simulink model "Bicycle_model"  (R2024b)
settings: Solver=VariableStepAuto  StartTime=0.0  StopTime=10  RelTol=1e-3
undefined symbols (not defined in the file): Af, Cd, Cl, Cr, g, GR, h_cg, Jf, Jr, M_sprung, Mv, r, rho, wb
libraries: simulink x1
settings Model: Creator=kanishka  LastModifiedBy=kanishka
settings DebuggingCC: AlgebraicLoopMsg=none

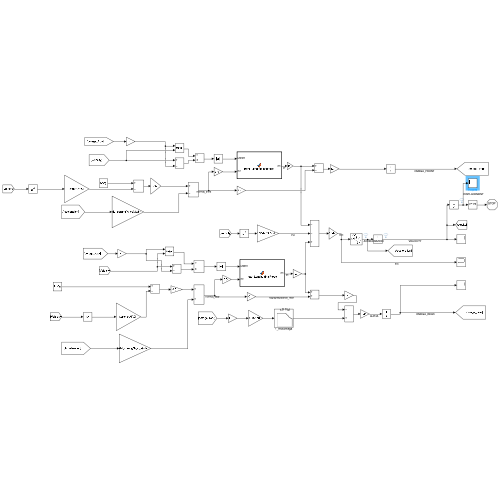
[thumbnail: Simulink's stored preview of the top-level diagram]
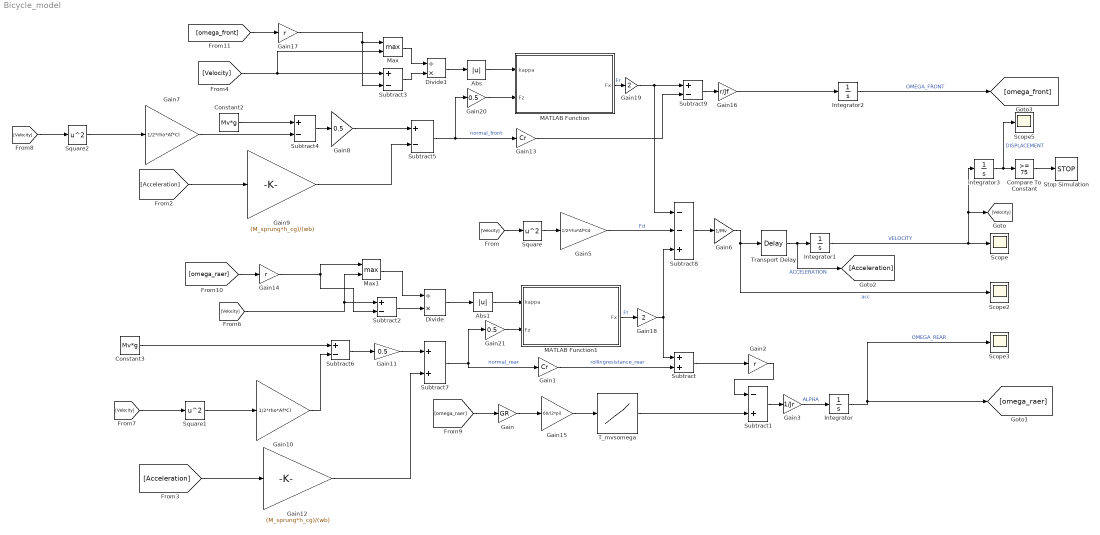
== system Bicycle_model ==
  Abs : Abs  SaturateOnIntegerOverflow=off
  Abs1 : Abs  SaturateOnIntegerOverflow=off
  Compare To Constant : simulink/Logic and Bit Operations/Compare To Constant  relop=>=  const=75  OutDataTypeStr=boolean
  Constant2 : Constant  Value=Mv*g
  Constant3 : Constant  Value=Mv*g
  Divide : Product  Inputs=/*
  Divide1 : Product  Inputs=/*
  Gain : Gain  Gain=GR
  Gain1 : Gain  Gain=Cr
  Gain10 : Gain  Gain=1/2*rho*Af*Cl
  Gain{8,11,20..21} (4 alike) : Gain  Gain=0.5
  Gain12 : Gain  Gain=(M_sprung*h_cg)/(wb)
  Gain13 : Gain  Gain=Cr
  Gain14 : Gain  Gain=r
  Gain15 : Gain  Gain=60/(2*pi)
  Gain16 : Gain  Gain=r/Jf
  Gain17 : Gain  Gain=r
  Gain18 : Gain  Gain=2
  Gain19 : Gain  Gain=2
  Gain2 : Gain  Gain=r
  Gain3 : Gain  Gain=1/Jr
  Gain5 : Gain  Gain=1/2*rho*Af*Cd
  Gain6 : Gain  Gain=1/Mv
  Gain7 : Gain  Gain=1/2*rho*Af*Cl
  Gain9 : Gain  Gain=(M_sprung*h_cg)/(wb)
  Integrator : Integrator  InitialCondition=0.0038455666
  Integrator1 : Integrator  InitialCondition=0.001
  Integrator2 : Integrator  InitialCondition=0.003457549
  Integrator3 : Integrator
  MATLAB Function : MATLAB Function  TreatAsAtomicUnit=on
  MATLAB Function1 : MATLAB Function  TreatAsAtomicUnit=on
  Max : MinMax  Function=max  Inputs=2
  Max1 : MinMax  Function=max  Inputs=2
  Scope{,2..3,5} (4 alike) : Scope
  Square : Math  Operator=square
  Square1 : Math  Operator=square
  Square2 : Math  Operator=square
  Stop Simulation : Stop
  Subtract : Sum
  Subtract1 : Sum  Inputs=-+
  Subtract{2..6,9} (6 alike) : Sum  Inputs=+-
  Subtract7 : Sum
  Subtract8 : Sum  Inputs=--+
  T_mvsomega : Lookup_n-D  NumberOfTableDimensions=1  BreakpointsForDimension1=[1, 3183, 3400, 3600, 3800, 4000, 4200, 4400, 4600, 4800, 5000, 5200, 5400, 5500, 5500.01] ;  Table=[240, 240, 224.653, 212.160, 200.988, 190.985, 181.818, 173.376, 165.571 ,158.408 ,152.788 ,147.016 ,141.381 ,138.991, 0]  InternalRulePriority=Speed  RndMeth=Simplest
  Transport Delay : TransportDelay  DelayTime=0.001  InitialOutput=0.85*g
  wires:
  Subtract4/1 -> Gain8/1
  Gain7/1 -> Subtract4/2
  Gain9/1 -> Subtract5/2
  Gain8/1 -> Subtract5/1
  Constant2/1 -> Subtract4/1
  Subtract5/1 -> Gain20/1, Gain13/1  "normal_front"
  Gain11/1 -> Subtract7/1
  Gain10/1 -> Subtract6/2
  Gain12/1 -> Subtract7/2
  Subtract6/1 -> Gain11/1
  Constant3/1 -> Subtract6/1
  Subtract7/1 -> Gain21/1, Gain1/1  "normal_rear"
  MATLAB Function1/1(Fx) -> Gain18/1  "Ft"
  Gain1/1 -> Subtract/2  "rollingresistance_rear"
  Subtract/1 -> Gain2/1
  Gain2/1 -> Subtract1/1
  Subtract1/1 -> Gain3/1
  Gain3/1 -> Integrator/1  "ALPHA"
  Integrator/1 -> Scope3/1, [omega_raer]  "OMEGA_REAR"
  Gain5/1 -> Subtract8/2  "Fd"
  Subtract8/1 -> Gain6/1
  Integrator1/1 -> Integrator3/1, [Velocity], Scope/1  "VELOCITY"
  Square/1 -> Gain5/1
  Gain6/1 -> Scope2/1, Transport Delay/1  "acc"
  [Velocity] -> Square/1
  [Acceleration] -> Gain9/1
  [Acceleration] -> Gain12/1
  [Velocity] -> Subtract3/1, Max/2
  [Velocity] -> Subtract2/1, Max1/2
  Square1/1 -> Gain10/1
  [Velocity] -> Square1/1
  [Velocity] -> Square2/1
  Square2/1 -> Gain7/1
  [omega_raer] -> Gain14/1
  Integrator3/1 -> Scope5/1, Compare To Constant/1  "DISPLACEMENT"
  Compare To Constant/1 -> Stop Simulation/1
  [omega_raer] -> Gain/1
  T_mvsomega/1 -> Subtract1/2
  Gain/1 -> Gain15/1
  Gain13/1 -> Subtract9/2
  Gain15/1 -> T_mvsomega/1
  Subtract9/1 -> Gain16/1
  Gain16/1 -> Integrator2/1
  Integrator2/1 -> [omega_front]  "OMEGA_FRONT"
  [omega_front] -> Gain17/1
  Subtract3/1 -> Divide1/2
  Subtract2/1 -> Divide/2
  Gain17/1 -> Subtract3/2, Max/1
  Max1/1 -> Divide/1
  Gain14/1 -> Subtract2/2, Max1/1
  Max/1 -> Divide1/1
  Transport Delay/1 -> [Acceleration], Integrator1/1  "ACCELERATION"
  Gain18/1 -> Subtract/1, Subtract8/3
  Gain19/1 -> Subtract8/1, Subtract9/1
  MATLAB Function/1(Fx) -> Gain19/1  "Fr"
  Divide1/1 -> Abs/1
  Divide/1 -> Abs1/1
  Abs/1 -> MATLAB Function/1(kappa)
  Gain20/1 -> MATLAB Function/2(Fz)
  Abs1/1 -> MATLAB Function1/1(kappa)
  Gain21/1 -> MATLAB Function1/2(Fz)

== matlab function Bicycle_model/MATLAB Function ==
  data: kappa input; Fz input; Fx output
function Fx = front_LongitudinalForce(kappa, Fz)
LFZO                         = 1 ;                
LCX                          = 1 ;                
LMUX                         = 1 ;                
LEX                          = 1 ;                
LKX                          = 1 ;                
LHX                          = 1 ;                
LVX                          = 1 ;                
PCX1                         = 1.5767 ;           
PDX1                         = 2.3195 ;           
PDX2                         = -0.013452  ;       
PEX1                         = -3.637e-13 ;       
PEX2                         = -0.28217   ;       
PEX3                         = -0.6       ;       
PEX4                         = 0.9        ;       
PKX1                         = 40.5424    ;       
PKX2                         = 29.9974    ;       
PKX3                         = -1.0517    ;       
PHX1                         = 0.0004551  ;       
PHX2                         = 0.0029521  ;       
PVX1                         = -0.023894  ;       
PVX2                         = -0.1       ;       

Fz0 = 1054;                  
dfz = (Fz - LFZO*Fz0) /(LFZO*Fz0);


mu_x = (PDX1 + PDX2 * dfz)* LMUX;


Dx = mu_x * Fz;

SHx = (PHX1 + PHX2 * dfz) * LHX;
Cx = PCX1 * LCX;
kappa_x = kappa + SHx;


Ex = (PEX1 + PEX2 * dfz + PEX3 * dfz^2) * (1 - PEX4 * sign(kappa_x)) * LEX;


Kx = Fz * (PKX1 + PKX2 * dfz) * exp(PKX3 * dfz) * LKX;


Bx = Kx / (Cx * Dx);


SVx = Fz * (PVX1 + PVX2 * dfz) * LVX * LMUX;





Fx0 = Dx * sin(Cx * atan(Bx * kappa_x - Ex * (Bx * kappa_x - atan(Bx * kappa_x)))) + SVx;


Fx = Fx0;

== matlab function Bicycle_model/MATLAB Function1 ==
  data: kappa input; Fz input; Fx output
function Fx =rear_LongitudinalForce(kappa, Fz)
LFZO                         = 1 ;                
LCX                          = 1 ;                
LMUX                         = 1 ;                
LEX                          = 1 ;                
LKX                          = 1 ;                
LHX                          = 1 ;                
LVX                          = 1 ;                
PCX1                         = 1.5767 ;           
PDX1                         = 2.3195 ;           
PDX2                         = -0.013452  ;       
PEX1                         = -3.637e-13 ;       
PEX2                         = -0.28217   ;       
PEX3                         = -0.6       ;       
PEX4                         = 0.9        ;       
PKX1                         = 40.5424    ;       
PKX2                         = 29.9974    ;       
PKX3                         = -1.0517    ;       
PHX1                         = 0.0004551  ;       
PHX2                         = 0.0029521  ;       
PVX1                         = -0.023894  ;       
PVX2                         = -0.1       ;       

Fz0 = 1054;                  
dfz = (Fz - LFZO*Fz0) /(LFZO*Fz0);


mu_x = (PDX1 + PDX2 * dfz)* LMUX;


Dx = mu_x * Fz;

SHx = (PHX1 + PHX2 * dfz) * LHX;
Cx = PCX1 * LCX;
kappa_x = kappa + SHx;


Ex = (PEX1 + PEX2 * dfz + PEX3 * dfz^2) * (1 - PEX4 * sign(kappa_x)) * LEX;


Kx = Fz * (PKX1 + PKX2 * dfz) * exp(PKX3 * dfz) * LKX;


Bx = Kx / (Cx * Dx);


SVx = Fz * (PVX1 + PVX2 * dfz) * LVX * LMUX;





Fx0 = Dx * sin(Cx * atan(Bx * kappa_x - Ex * (Bx * kappa_x - atan(Bx * kappa_x)))) + SVx;


Fx = Fx0;
